simulink model "PMSM_Demo"  (R2019b)
settings: Solver=FixedStepDiscrete  StartTime=0.0  StopTime=Inf  FixedStep=1000e-6  RelTol=1e-3  EnableMultiTasking=on
PreLoadFcn:
  | run('PMSM_Demo_ini.m');
PostLoadFcn:
  | , if any(exist('dsrtsu_mdlpostloadfcn', 'file') ~= 0), dsrtsu_mdlpostloadfcn('Execute', bdroot); end,
InitFcn:
  | , if any(exist('rtifpga_mdlclblib', 'file') ~= 0), rtifpga_mdlclblib('Init', bdroot); end,
values from neighbouring files (symbols this model uses):
  Const_Id_Fieldweakening = 0    [PMSM_Demo_ini.m]
  Const_Ld_Stator = L    (= 0.0004)    [PMSM_Demo_ini.m]
  Const_Lq_Stator = L    (= 0.0004)    [PMSM_Demo_ini.m]
  Const_PolePairs = PolePairs    (= 4)    [PMSM_Demo_ini.m]
  Const_Psi = Psi    (= 0.017)    [PMSM_Demo_ini.m]
  PMSM_Ctrl_Ctrl_mode_SW = 3    [PMSM_Demo_ini.m]
  PMSM_Ctrl_fRS_Set = 0    [PMSM_Demo_ini.m]
  PMSM_Ctrl_i_d_Set = 0    [PMSM_Demo_ini.m]
  PMSM_Ctrl_i_d_Stroke = 0    [PMSM_Demo_ini.m]
  PMSM_Ctrl_i_q_Set = 0    [PMSM_Demo_ini.m]
  PMSM_Ctrl_i_q_Stroke = 0    [PMSM_Demo_ini.m]
  PMSM_Ctrl_Ki_id = KI_i    (= 3595.02029348)    [PMSM_Demo_ini.m]
  PMSM_Ctrl_Ki_iq = KI_i    (= 3595.02029348)    [PMSM_Demo_ini.m]
  PMSM_Ctrl_Ki_n = KI_n    (= 50.0861118327)    [PMSM_Demo_ini.m]
  PMSM_Ctrl_Kp_id = KP_i    (= 1.54995705396)    [PMSM_Demo_ini.m]
  PMSM_Ctrl_Kp_iq = KP_i    (= 1.54995705396)    [PMSM_Demo_ini.m]
  PMSM_Ctrl_Kp_n = KP_n    (= 0.0775235575931)    [PMSM_Demo_ini.m]
  PMSM_Ctrl_Limit_iq = IQ_MAX    (= 10.6)    [PMSM_Demo_ini.m]
  PMSM_Ctrl_load_torque = 0    [PMSM_Demo_ini.m]
  PMSM_Ctrl_n_Limit = N_MAX    (= 3000)    [PMSM_Demo_ini.m]
  PMSM_Ctrl_n_Set = 0    [PMSM_Demo_ini.m]
  PMSM_Ctrl_n_Stroke = 0    [PMSM_Demo_ini.m]
  PMSM_Ctrl_Pos_Src = 1    [PMSM_Demo_ini.m]
  PMSM_Ctrl_TF_Id = TF_i    (= 7.95774715459e-05)    [PMSM_Demo_ini.m]
  PMSM_Ctrl_TF_Iq = TF_i    (= 7.95774715459e-05)    [PMSM_Demo_ini.m]
  PMSM_Ctrl_TF_n = TF_n    (= 0.00106103295395)    [PMSM_Demo_ini.m]
  PMSM_Ctrl_theta_offset = 0.5    [PMSM_Demo_ini.m]
  PMSM_Ctrl_v_d_Set = 0    [PMSM_Demo_ini.m]
  PMSM_Ctrl_V_DCLink_Limit = UD    (= 15)    [PMSM_Demo_ini.m]
  PMSM_Ctrl_v_q_Set = 0    [PMSM_Demo_ini.m]
  PMSM_Ctrl_Vel_Src = 4    [PMSM_Demo_ini.m]
  SW_Fieldweakening = 2    [PMSM_Demo_ini.m]
  T_PWM = 50e-6    (= 5e-05)    [PMSM_Demo_ini.m]
undefined symbols (not defined in the file or in its folder): clock, Newton, Raphson, rpm_to_rad, s
libraries: simulink x37, rti1202lib_adc_class1 x8, dsextras x4, rtiemclib x4, rti1202lib_dio_class1 x3, ASM_ElectricComponents_lib x2, ASM_Utils_lib x1, rti1202lib_base x1
(part 4 of 4)

== system PMSM_Demo/Control/Controller/PMSM_CONTROLLER/current_controller/current_transformation_disp ==
  in1 : Inport
  demux : Demux  Outputs=2
  transf : Subsystem
      settings: AttributesFormatString=clarke
  out1 : Outport  VectorParamsAs1DForOutWhenUnconnected=off
  out2 : Outport  Port=2  VectorParamsAs1DForOutWhenUnconnected=off
  wires:
  in1/1 -> transf/1(in)
  transf/1(out) -> demux/1
  demux/1 -> out1/1
  demux/2 -> out2/1

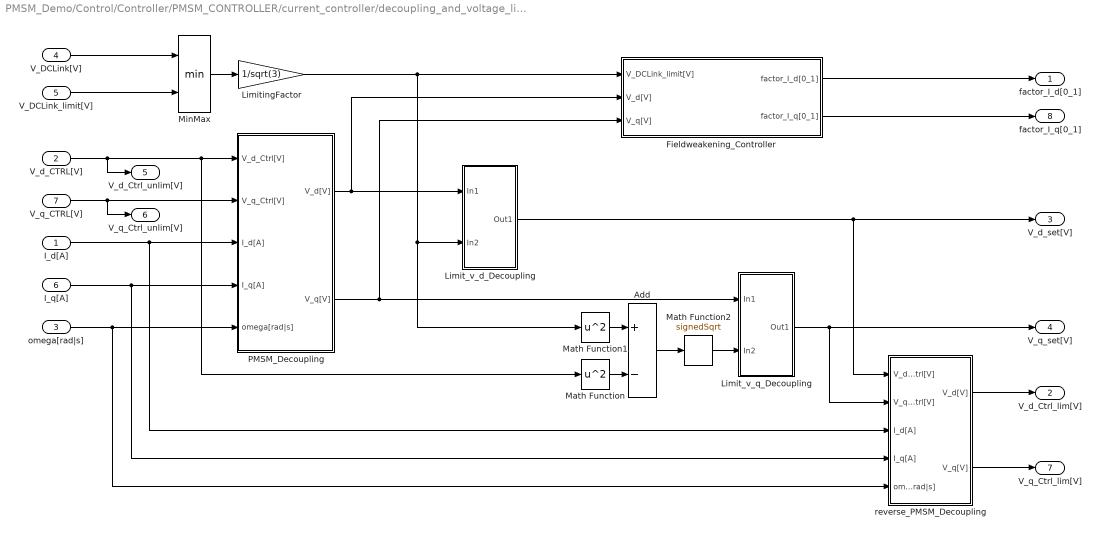
== system PMSM_Demo/Control/Controller/PMSM_CONTROLLER/current_controller/decoupling_and_voltage_limitation ==
  I_d[A] : Inport
  V_d_CTRL[V] : Inport  Port=2
  omega[rad|s] : Inport  Port=3
  V_DCLink[V] : Inport  Port=4
  V_DCLink_limit[V] : Inport  Port=5
  I_q[A] : Inport  Port=6
  V_q_CTRL[V] : Inport  Port=7
  Add : Sum  Inputs=+-
  Fieldweakening_Controller : Subsystem
  Limit_v_d_Decoupling : Subsystem
      mask Display: plot([0.15 0.85],[.5 .5],[.5 .5],[0.05 0.95],0.15+0.7*[0 .25 .75 1],0.05+0.9*[.25 .25 .75 .75]);
  Limit_v_q_Decoupling : Subsystem
      mask Display: plot([0.15 0.85],[.5 .5],[.5 .5],[0.05 0.95],0.15+0.7*[0 .25 .75 1],0.05+0.9*[.25 .25 .75 .75]);
  LimitingFactor : Gain  Gain=1/sqrt(3)
  Math Function : Math  Operator=square  SaturateOnIntegerOverflow=on
  Math Function1 : Math  Operator=square  SaturateOnIntegerOverflow=on
  Math Function2 : Sqrt  Operator=signedSqrt  AlgorithmType=Newton-Raphson  SaturateOnIntegerOverflow=on
  MinMax : MinMax  Inputs=2
  PMSM_Decoupling : Subsystem
  reverse_PMSM_Decoupling : Subsystem
  factor_I_d[0_1] : Outport  VectorParamsAs1DForOutWhenUnconnected=off
  V_d_Ctrl_lim[V] : Outport  Port=2  VectorParamsAs1DForOutWhenUnconnected=off
  V_d_set[V] : Outport  Port=3  VectorParamsAs1DForOutWhenUnconnected=off
  V_q_set[V] : Outport  Port=4  VectorParamsAs1DForOutWhenUnconnected=off
  V_d_Ctrl_unlim[V] : Outport  Port=5  VectorParamsAs1DForOutWhenUnconnected=off
  V_q_Ctrl_unlim[V] : Outport  Port=6  VectorParamsAs1DForOutWhenUnconnected=off
  V_q_Ctrl_lim[V] : Outport  Port=7  VectorParamsAs1DForOutWhenUnconnected=off
  factor_I_q[0_1] : Outport  Port=8  VectorParamsAs1DForOutWhenUnconnected=off
  wires:
  Fieldweakening_Controller/2(factor_I_q[0_1]) -> factor_I_q[0_1]/1
  Fieldweakening_Controller/1(factor_I_d[0_1]) -> factor_I_d[0_1]/1
  Math Function2/1 -> Limit_v_q_Decoupling/2(In2)
  V_DCLink_limit[V]/1 -> MinMax/2
  Limit_v_q_Decoupling/1(Out1) -> reverse_PMSM_Decoupling/2(V_q_Ctrl[V]), V_q_set[V]/1
  Limit_v_d_Decoupling/1(Out1) -> reverse_PMSM_Decoupling/1(V_d_Ctrl[V]), V_d_set[V]/1
  reverse_PMSM_Decoupling/2(V_q[V]) -> V_q_Ctrl_lim[V]/1
  reverse_PMSM_Decoupling/1(V_d[V]) -> V_d_Ctrl_lim[V]/1
  PMSM_Decoupling/2(V_q[V]) -> Limit_v_q_Decoupling/1(In1), Fieldweakening_Controller/3(V_q[V])
  Add/1 -> Math Function2/1
  Math Function/1 -> Add/2
  Math Function1/1 -> Add/1
  LimitingFactor/1 -> Math Function1/1, Limit_v_d_Decoupling/2(In2), Fieldweakening_Controller/1(V_DCLink_limit[V])
  omega[rad|s]/1 -> reverse_PMSM_Decoupling/5(omega[rad|s]), PMSM_Decoupling/5(omega[rad|s])
  PMSM_Decoupling/1(V_d[V]) -> Limit_v_d_Decoupling/1(In1), Fieldweakening_Controller/2(V_d[V])
  I_d[A]/1 -> reverse_PMSM_Decoupling/3(I_d[A]), PMSM_Decoupling/3(I_d[A])
  I_q[A]/1 -> reverse_PMSM_Decoupling/4(I_q[A]), PMSM_Decoupling/4(I_q[A])
  V_d_CTRL[V]/1 -> Math Function/1, PMSM_Decoupling/1(V_d_Ctrl[V]), V_d_Ctrl_unlim[V]/1
  V_q_CTRL[V]/1 -> PMSM_Decoupling/2(V_q_Ctrl[V]), V_q_Ctrl_unlim[V]/1
  V_DCLink[V]/1 -> MinMax/1
  MinMax/1 -> LimitingFactor/1

== system PMSM_Demo/Control/Controller/PMSM_CONTROLLER/current_controller/manip_i_d ==
  Factor_i_d[0_1] : Inport
  I_d_Set[A] : Inport  Port=2
  SW : Inport  Port=3
  Multiport Switch : MultiPortSwitch
  factor_id : Product  RndMeth=Zero
  Out1 : Outport  VectorParamsAs1DForOutWhenUnconnected=off
  wires:
  factor_id/1 -> Multiport Switch/2
  Factor_i_d[0_1]/1 -> factor_id/1
  Multiport Switch/1 -> Out1/1
  SW/1 -> Multiport Switch/1
  I_d_Set[A]/1 -> Multiport Switch/4, Multiport Switch/3, factor_id/2

== system PMSM_Demo/Control/Controller/PMSM_CONTROLLER/current_controller/manip_i_q ==
  SW : Inport
  I_q_Set[A] : Inport  Port=2
  Factor_i_q[0_1] : Inport  Port=3
  Multiport Switch : MultiPortSwitch
  factor_id : Product  RndMeth=Zero
  Out1 : Outport  VectorParamsAs1DForOutWhenUnconnected=off
  wires:
  factor_id/1 -> Multiport Switch/2
  Factor_i_q[0_1]/1 -> factor_id/1
  I_q_Set[A]/1 -> Multiport Switch/4, Multiport Switch/3, factor_id/2
  SW/1 -> Multiport Switch/1
  Multiport Switch/1 -> Out1/1

== system PMSM_Demo/Control/Controller/PMSM_CONTROLLER/i_set_source_SW/Limit_id_Set ==
  In1 : Inport
  In2 : Inport  Port=2
  Saturation Dynamic : simulink/Discontinuities/Saturation Dynamic  OutMin=[]  OutMax=[]  OutDataTypeStr=Inherit: Same as second input  OutDataType=sfix(16)  OutScaling=2^-10  DoSatur=off
  inv : Gain  Gain=-1
  Out1 : Outport  VectorParamsAs1DForOutWhenUnconnected=off
  wires:
  inv/1 -> Saturation Dynamic/3
  In2/1 -> Saturation Dynamic/1, inv/1
  In1/1 -> Saturation Dynamic/2
  Saturation Dynamic/1 -> Out1/1

== system PMSM_Demo/Control/Controller/PMSM_CONTROLLER/i_set_source_SW/Limit_iq_Set ==
  In1 : Inport
  In2 : Inport  Port=2
  Saturation Dynamic : simulink/Discontinuities/Saturation Dynamic  OutMin=[]  OutMax=[]  OutDataTypeStr=Inherit: Same as second input  OutDataType=sfix(16)  OutScaling=2^-10  DoSatur=off
  inv : Gain  Gain=-1
  Out1 : Outport  VectorParamsAs1DForOutWhenUnconnected=off
  wires:
  Saturation Dynamic/1 -> Out1/1
  In1/1 -> Saturation Dynamic/2
  In2/1 -> inv/1, Saturation Dynamic/1
  inv/1 -> Saturation Dynamic/3

== system PMSM_Demo/Control/Controller/PMSM_CONTROLLER/speed_controller/DISCRETE_PT1 ==
  Reset[0|1] : Inport
  In : Inport  Port=2
  K : Inport  Port=3
  T[s] : Inport  Port=4
  T_Sample[s] : Inport  Port=5
  1|FilterTime : Product  Inputs=*/  SaturateOnIntegerOverflow=on  InputSameDT=on  OutDataTypeStr=Inherit: Same as first input
  Proportional : Product  Inputs=**  SaturateOnIntegerOverflow=on  InputSameDT=on  OutDataTypeStr=Inherit: Same as first input
  Sum : Sum  Inputs=-+|  SaturateOnIntegerOverflow=on  InputSameDT=on  OutDataTypeStr=Inherit: Same as first input
  Unit Delay : UnitDelay  SampleTime=-1  HasFrameUpgradeWarning=on
  discrete_Integrator_Init : Subsystem  mask(DISCRETE_INTEGRATOR){upper_limit=upper_limit_int, lower_limit=lower_limit_int, ASMProperties=struct('Name','discrete_integrator','Version','1.0','Library','ASM_ElectricComponents_lib')}
      mask prompts: upper_limit "upper limit"; lower_limit "lower limit"
      mask help: (c) Copyright 2007, dSPACE GmbH. All rights reserved.
      mask Help: eval(['asm_modelhelp(gcbh)'])
  zero : Constant  Value=0  SampleTime=-1
  Out : Outport  VectorParamsAs1DForOutWhenUnconnected=off
  wires:
  In/1 -> Proportional/1
  Sum/1 -> discrete_Integrator_Init/2(In)
  K/1 -> Proportional/2
  Proportional/1 -> Sum/2
  discrete_Integrator_Init/1(Out) -> 1|FilterTime/1
  1|FilterTime/1 -> Out/1, Unit Delay/1
  Unit Delay/1 -> Sum/1
  T[s]/1 -> 1|FilterTime/2
  Reset[0|1]/1 -> discrete_Integrator_Init/1(Reset[0|1])
  T_Sample[s]/1 -> discrete_Integrator_Init/4(T_Sample[s])
  zero/1 -> discrete_Integrator_Init/3(Initial)

== system PMSM_Demo/Control/Controller/PMSM_CONTROLLER/speed_controller/DISCRETE_PT1_SET ==
  Reset[0|1] : Inport
  In : Inport  Port=2
  K : Inport  Port=3
  T[s] : Inport  Port=4
  T_Sample[s] : Inport  Port=5
  1|FilterTime : Product  Inputs=*/  SaturateOnIntegerOverflow=on  InputSameDT=on  OutDataTypeStr=Inherit: Same as first input
  Proportional : Product  Inputs=**  SaturateOnIntegerOverflow=on  InputSameDT=on  OutDataTypeStr=Inherit: Same as first input
  Sum : Sum  Inputs=-+|  SaturateOnIntegerOverflow=on  InputSameDT=on  OutDataTypeStr=Inherit: Same as first input
  Unit Delay : UnitDelay  SampleTime=-1  HasFrameUpgradeWarning=on
  discrete_Integrator_Init : Subsystem  mask(DISCRETE_INTEGRATOR){upper_limit=upper_limit_int, lower_limit=lower_limit_int, ASMProperties=struct('Name','discrete_integrator','Version','1.0','Library','ASM_ElectricComponents_lib')}
      mask prompts: upper_limit "upper limit"; lower_limit "lower limit"
      mask help: (c) Copyright 2007, dSPACE GmbH. All rights reserved.
      mask Help: eval(['asm_modelhelp(gcbh)'])
  zero : Constant  Value=0  SampleTime=-1
  Out : Outport  VectorParamsAs1DForOutWhenUnconnected=off
  wires:
  zero/1 -> discrete_Integrator_Init/3(Initial)
  T_Sample[s]/1 -> discrete_Integrator_Init/4(T_Sample[s])
  Reset[0|1]/1 -> discrete_Integrator_Init/1(Reset[0|1])
  T[s]/1 -> 1|FilterTime/2
  Unit Delay/1 -> Sum/1
  1|FilterTime/1 -> Unit Delay/1, Out/1
  discrete_Integrator_Init/1(Out) -> 1|FilterTime/1
  Proportional/1 -> Sum/2
  K/1 -> Proportional/2
  Sum/1 -> discrete_Integrator_Init/2(In)
  In/1 -> Proportional/1

== system PMSM_Demo/Control/Controller/PMSM_CONTROLLER/speed_controller/Limit_n_Set ==
  In1 : Inport
  In2 : Inport  Port=2
  Saturation Dynamic : simulink/Discontinuities/Saturation Dynamic  OutMin=[]  OutMax=[]  OutDataTypeStr=Inherit: Same as second input  OutDataType=sfix(16)  OutScaling=2^-10  DoSatur=off
  inv : Gain  Gain=-1
  Out1 : Outport  VectorParamsAs1DForOutWhenUnconnected=off
  wires:
  inv/1 -> Saturation Dynamic/3
  In2/1 -> Saturation Dynamic/1, inv/1
  In1/1 -> Saturation Dynamic/2
  Saturation Dynamic/1 -> Out1/1

== system PMSM_Demo/Control/Controller/PMSM_CONTROLLER/speed_controller/PI_CONTROLLER ==
  ActualValue : Inport
  RefValue : Inport  Port=2
  Kp : Inport  Port=3
  Ki : Inport  Port=4
  Limit_up : Inport  Port=5
  Limit_lo : Inport  Port=6
  T_Sample[s] : Inport  Port=7
  Product : Product  RndMeth=Zero
  Product1 : Product  RndMeth=Zero
  Product2 : Product  RndMeth=Zero
  Saturation Dynamic : simulink/Discontinuities/Saturation Dynamic  OutMin=[]  OutMax=[]  OutDataTypeStr=Inherit: Same as second input  OutDataType=sfix(16)  OutScaling=2^-10  DoSatur=off
  Sum : Sum  Inputs=+++  SaturateOnIntegerOverflow=on
  Sum1 : Sum  Inputs=+-  SaturateOnIntegerOverflow=on
  Sum2 : Sum  Inputs=-+|  SaturateOnIntegerOverflow=on
  Unit Delay : UnitDelay  SampleTime=-1  HasFrameUpgradeWarning=on
  y : Outport  VectorParamsAs1DForOutWhenUnconnected=off
  wires:
  Limit_lo/1 -> Saturation Dynamic/3
  Limit_up/1 -> Saturation Dynamic/1
  Sum/1 -> Saturation Dynamic/2
  Sum1/1 -> Product1/2, Product2/1  "error"
  RefValue/1 -> Sum1/1
  ActualValue/1 -> Sum1/2
  Product1/1 -> Sum/1, Sum2/1
  Product/1 -> Sum/2  "integral"
  Saturation Dynamic/1 -> Sum2/2, y/1
  Product2/1 -> Product/1
  Unit Delay/1 -> Sum/3
  Sum2/1 -> Unit Delay/1
  T_Sample[s]/1 -> Product/2
  Kp/1 -> Product1/1
  Ki/1 -> Product2/2

== system PMSM_Demo/Control/Controller/PMSM_CONTROLLER/speed_controller/SignalCollector ==
  n_Limit[rpm] : Inport
  n[rpm] : Inport  Port=2
  n_Set[rpm] : Inport  Port=3
  Bus Creator : BusCreator  Inputs=3
  SignalBus : Outport  VectorParamsAs1DForOutWhenUnconnected=off
  wires:
  n_Limit[rpm]/1 -> Bus Creator/3  "n_Limit[rpm]"
  Bus Creator/1 -> SignalBus/1  "SPEED_CONTROLLER"
  n_Set[rpm]/1 -> Bus Creator/2  "n_Set[rpm]"
  n[rpm]/1 -> Bus Creator/1  "n[rpm]"

== system PMSM_Demo/Control/Controller/PMSM_CONTROLLER/v_set_source_SW/Calc_Angle ==
  f_set[Hz] : Inport
  T_Sample[s] : Inport  Port=2
  DISCRETE_INTEGRATOR : Subsystem  mask(DISCRETE_INTEGRATOR){upper_limit=struct('v', 1e300), lower_limit=struct('v', -1e300), ASMProperties=struct('Name','DISCRETE_INTEGRATOR','Version','1.0','Library','ASM_ElectricComponents_lib')}
      mask prompts: upper_limit "upper limit"; lower_limit "lower limit"
      mask help: (c) Copyright 2007, dSPACE GmbH. All rights reserved.
      mask Help: eval(['asm_modelhelp(gcbh)'])
  Lim[0...2*pi] : Subsystem
  Reset[0|1] : Constant  Value=0
  "[rpm]2[rad|s]" : ASM_Utils_lib/UnitConversion/UnitConversion  Selection=rpm_to_rad/s
  torpm : Gain  Gain=60  SaturateOnIntegerOverflow=on  OutDataTypeStr=Inherit: Same as input  ParamDataTypeStr=Inherit: Same as input
  zero : Constant  Value=0
  theta[rad] : Outport  VectorParamsAs1DForOutWhenUnconnected=off
  wires:
  Lim[0...2*pi]/1(theta_lim) -> theta[rad]/1
  T_Sample[s]/1 -> DISCRETE_INTEGRATOR/4(T_Sample[s])
  torpm/1 -> "[rpm]2[rad|s]"/1
  Reset[0|1]/1 -> DISCRETE_INTEGRATOR/1(Reset[0|1])
  zero/1 -> DISCRETE_INTEGRATOR/3(Initial)
  DISCRETE_INTEGRATOR/1(Out) -> Lim[0...2*pi]/1(theta_unlim)
  f_set[Hz]/1 -> torpm/1
  "[rpm]2[rad|s]"/1 -> DISCRETE_INTEGRATOR/2(In)

== system PMSM_Demo/Control/Controller/PMSM_CONTROLLER/v_set_source_SW/Label_v_Stator[a;b;c][V] ==
  In : Inport
  Bus Creator : BusCreator  Inputs=3
  Demux : Demux  Outputs=3
  Out : Outport  VectorParamsAs1DForOutWhenUnconnected=off
  wires:
  In/1 -> Demux/1
  Bus Creator/1 -> Out/1
  Demux/1 -> Bus Creator/1  "V_a_Stator[V]"
  Demux/2 -> Bus Creator/2  "V_b_Stator[V]"
  Demux/3 -> Bus Creator/3  "V_c_Stator[V]"

== system PMSM_Demo/Control/Input/DISCRETE_PT1/discrete_Integrator_Init/only_rising_edge  ==
  In1 : Inport
  Compare To Constant1 : simulink/Logic and Bit Operations/Compare To Constant  relop===  const=0  OutDataTypeStr=uint8  ZeroCross=off
  Compare To Constant2 : simulink/Logic and Bit Operations/Compare To Constant  relop===  const=1  OutDataTypeStr=uint8  ZeroCross=off
  Logical Operator1 : Logic  AllPortsSameDT=off  OutDataTypeStr=boolean
  Unit Delay2 : UnitDelay  SampleTime=-1  HasFrameUpgradeWarning=on
  Out1 : Outport  VectorParamsAs1DForOutWhenUnconnected=off
  wires:
  Logical Operator1/1 -> Out1/1
  Compare To Constant2/1 -> Logical Operator1/2
  Compare To Constant1/1 -> Logical Operator1/1
  In1/1 -> Compare To Constant2/1, Unit Delay2/1
  Unit Delay2/1 -> Compare To Constant1/1

== system PMSM_Demo/RTI Data/RTI Data Store/RTI Data Store/RTI Data Store/RTI Data Store ==

== system PMSM_Demo/Control/Controller/PMSM_CONTROLLER/current_controller/DISCRETE_PT1/discrete_Integrator_Init ==
  Reset[0|1] : Inport
  In : Inport  Port=2
  Initial : Inport  Port=3
  T_Sample[s] : Inport  Port=4
  Add : Sum  Inputs=+++
  Compare To Constant : simulink/Logic and Bit Operations/Compare To Constant  relop===  const=0  OutDataTypeStr=uint8  ZeroCross=off
  Constant1 : Constant  Value=0
  Constant2 : Constant  Value=0
  Logical Operator : Logic  Operator=OR  AllPortsSameDT=off  OutDataTypeStr=boolean
  Product : Product  RndMeth=Zero
  Saturation : simulink/Discontinuities/Saturation Dynamic  OutMin=[]  OutMax=[]  OutDataTypeStr=Inherit: Same as second input  OutDataType=sfix(16)  OutScaling=2^-10  DoSatur=off
  Switch1 : Switch  Threshold=0.5
  Switch2 : Switch  Threshold=0.5
  Unit Delay : UnitDelay  SampleTime=-1  HasFrameUpgradeWarning=on
  Unit Delay1 : UnitDelay  SampleTime=-1  HasFrameUpgradeWarning=on
  lower_limit : Constant  Value=lower_limit.v
  "only_rising_edge " : Subsystem
  upper_limit : Constant  Value=upper_limit.v
  Out : Outport  VectorParamsAs1DForOutWhenUnconnected=off
  wires:
  Compare To Constant/1 -> Logical Operator/1
  Logical Operator/1 -> Switch1/2
  Unit Delay1/1 -> Compare To Constant/1
  "only_rising_edge "/1(Out1) -> Switch2/2, Logical Operator/2
  Constant1/1 -> Switch1/3
  Initial/1 -> Switch1/1
  Switch1/1 -> Add/1
  Unit Delay/1 -> Switch2/3
  Switch2/1 -> Add/3
  Constant2/1 -> Switch2/1
  In/1 -> Product/2
  Reset[0|1]/1 -> "only_rising_edge "/1(In1)
  Product/1 -> Add/2
  T_Sample[s]/1 -> Unit Delay1/1, Product/1
  Add/1 -> Saturation/2
  Saturation/1 -> Out/1, Unit Delay/1
  upper_limit/1 -> Saturation/1
  lower_limit/1 -> Saturation/3

== system PMSM_Demo/Control/Controller/PMSM_CONTROLLER/current_controller/DISCRETE_PT2/discrete_Integrator_Init ==
  Reset[0|1] : Inport
  In : Inport  Port=2
  Initial : Inport  Port=3
  T_Sample[s] : Inport  Port=4
  Add : Sum  Inputs=+++
  Compare To Constant : simulink/Logic and Bit Operations/Compare To Constant  relop===  const=0  OutDataTypeStr=uint8  ZeroCross=off
  Constant1 : Constant  Value=0
  Constant2 : Constant  Value=0
  Logical Operator : Logic  Operator=OR  AllPortsSameDT=off  OutDataTypeStr=boolean
  Product : Product  RndMeth=Zero
  Saturation : simulink/Discontinuities/Saturation Dynamic  OutMin=[]  OutMax=[]  OutDataTypeStr=Inherit: Same as second input  OutDataType=sfix(16)  OutScaling=2^-10  DoSatur=off
  Switch1 : Switch  Threshold=0.5
  Switch2 : Switch  Threshold=0.5
  Unit Delay : UnitDelay  SampleTime=-1  HasFrameUpgradeWarning=on
  Unit Delay1 : UnitDelay  SampleTime=-1  HasFrameUpgradeWarning=on
  lower_limit : Constant  Value=lower_limit.v
  "only_rising_edge " : Subsystem
  upper_limit : Constant  Value=upper_limit.v
  Out : Outport  VectorParamsAs1DForOutWhenUnconnected=off
  wires:
  lower_limit/1 -> Saturation/3
  upper_limit/1 -> Saturation/1
  Saturation/1 -> Unit Delay/1, Out/1
  Add/1 -> Saturation/2
  T_Sample[s]/1 -> Product/1, Unit Delay1/1
  Product/1 -> Add/2
  Reset[0|1]/1 -> "only_rising_edge "/1(In1)
  In/1 -> Product/2
  Constant2/1 -> Switch2/1
  Switch2/1 -> Add/3
  Unit Delay/1 -> Switch2/3
  Switch1/1 -> Add/1
  Initial/1 -> Switch1/1
  Constant1/1 -> Switch1/3
  "only_rising_edge "/1(Out1) -> Logical Operator/2, Switch2/2
  Unit Delay1/1 -> Compare To Constant/1
  Logical Operator/1 -> Switch1/2
  Compare To Constant/1 -> Logical Operator/1

== system PMSM_Demo/Control/Controller/PMSM_CONTROLLER/current_controller/current transformation/transf ==
  in : Inport
  Demux : Demux  Outputs=[3 1]
  Demux1 : Demux  Outputs=2
  Gain1 : Gain  Gain=[[2/3 -1/3 -1/3]*transffactor;[0 sqrt(3)/3 -sqrt(3)/3]*transffactor]  Multiplication=Matrix(K*u)  SaturateOnIntegerOverflow=on  OutDataTypeStr=Inherit: Same as input  ParamDataTypeStr=Inherit: Same as input
  Mux : Mux  Inputs=2
  Product{1..4} (4 alike) : Product  SaturateOnIntegerOverflow=on  OutDataTypeStr=Inherit: Same as first input
  Sum : Sum  SaturateOnIntegerOverflow=on
  Sum1 : Sum  SaturateOnIntegerOverflow=on
  cos : Fcn  Expr=cos(u)
  inv : Gain  Gain=-1  SaturateOnIntegerOverflow=on  OutDataTypeStr=Inherit: Same as input  ParamDataTypeStr=Inherit: Same as input
  sin : Fcn  Expr=sin(u)
  out : Outport  VectorParamsAs1DForOutWhenUnconnected=off
  wires:
  Mux/1 -> out/1
  in/1 -> Demux/1
  Demux/1 -> Gain1/1
  sin/1 -> inv/1, Product2/2
  Product3/1 -> Sum/1
  Product4/1 -> Sum/2
  Product2/1 -> Sum1/2
  Product1/1 -> Sum1/1
  Sum1/1 -> Mux/1
  Sum/1 -> Mux/2
  Demux/2 -> sin/1, cos/1
  cos/1 -> Product1/2, Product4/2
  inv/1 -> Product3/2
  Demux1/1 -> Product1/1, Product3/1
  Gain1/1 -> Demux1/1
  Demux1/2 -> Product2/1, Product4/1

== system PMSM_Demo/Control/Controller/PMSM_CONTROLLER/current_controller/current_transformation_disp/transf ==
  in : Inport
  Gain1 : Gain  Gain=[[2/3 -1/3 -1/3]*1;[0 sqrt(3)/3 -sqrt(3)/3]*1]  Multiplication=Matrix(K*u)  SaturateOnIntegerOverflow=on  OutDataTypeStr=Inherit: Same as input  ParamDataTypeStr=Inherit: Same as input
  out : Outport  VectorParamsAs1DForOutWhenUnconnected=off
  wires:
  in/1 -> Gain1/1
  Gain1/1 -> out/1

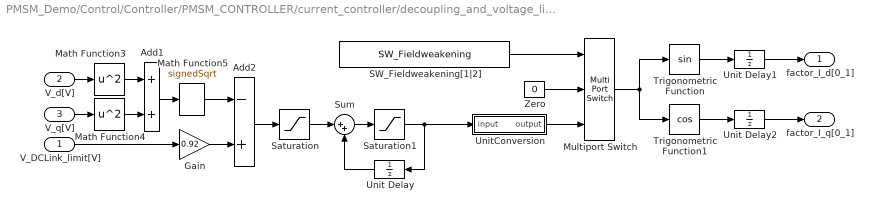
== system PMSM_Demo/Control/Controller/PMSM_CONTROLLER/current_controller/decoupling_and_voltage_limitation/Fieldweakening_Controller ==
  V_DCLink_limit[V] : Inport
  V_d[V] : Inport  Port=2
  V_q[V] : Inport  Port=3
  Add1 : Sum
  Add2 : Sum  Inputs=-+
  Gain : Gain  Gain=0.92
  Math Function3 : Math  Operator=square  SaturateOnIntegerOverflow=on
  Math Function4 : Math  Operator=square  SaturateOnIntegerOverflow=on
  Math Function5 : Sqrt  Operator=signedSqrt  AlgorithmType=Newton-Raphson  SaturateOnIntegerOverflow=on
  Multiport Switch : MultiPortSwitch  Inputs=2
  SW_Fieldweakening[1|2] : Constant  Value=SW_Fieldweakening
  Saturation : Saturate  UpperLimit=0.2  LowerLimit=-0.2
  Saturation1 : Saturate  UpperLimit=0  LowerLimit=-50
  Sum : Sum  Inputs=|++
  Trigonometric Function : Trigonometry
  Trigonometric Function1 : Trigonometry  Operator=cos
  Unit Delay : UnitDelay  SampleTime=-1  HasFrameUpgradeWarning=on
  Unit Delay1 : UnitDelay  SampleTime=-1  HasFrameUpgradeWarning=on
  Unit Delay2 : UnitDelay  SampleTime=-1  HasFrameUpgradeWarning=on
  UnitConversion : Subsystem  mask{Selection=deg_to_rad}
      mask prompts: Selection "Conversion:"
      mask init:
      | if(~exist('DS_CONTROLDESK_EVALUATION'))
      |     
      |   switch Selection
      |       
      |     case 'none'
      |       Offset = 0; Gain = 1; Unit1 = ''; Unit2 = '';      
      |     case 'bar_to_Pa'
      |       Offset = 0; Gain = 100000; Unit1 = 'bar'; Unit2 = 'Pa';
      |     case 'rad_to_deg'
      |       Offset = 0; Gain = 180/pi; Unit1 = 'rad'; Unit2 = 'deg';
      |     case 'deg_to_rad'
      |       Offset = 0; Gain = pi/180; Unit1 = 'deg'; Unit2 = 'rad';
      |     case 'degC_to_K'
      |       Offset = 273; Gain = 1; Unit1 = 'degC'; Unit2 = 'K';
      |     case 'K_to_degC'
      |       Offset = -273; Gain = 1; Unit1 = 'K'; Unit2 = 'degC';      
      |     case 'km/h_to_m/s'
      |       Offset = 0; Gain = 1/3.6; Unit1 = 'km|h'; Unit2 = 'm|s';
      |     case 'kg/h_to_kg/s'
      |       Offset = 0; Gain = 1/3600; Unit1 = 'kg|h'; Unit2 = 'kg|s';
      |     case 'kg/s_to_kg/h'
      |       Offset = 0; Gain = 3600; Unit1 = 'kg|s'; Unit2 = 'kg|h';
      |     case 'm/s_to_km/h'
      |       Offset = 0; Gain = 3.6; Unit1 = 'm|s'; Unit2 = 'km|h';
      |     case 'mm_to_m'
      |       Offset = 0; Gain = 1/1000; Unit1 = 'mm'; Unit2 = 'm';
      |     case 'mm_to_cm'
      |       Offset = 0; Gain = 1/10; Unit1 = 'mm'; Unit2 = 'cm';
      |     case 'm_to_mm'
      |       Offset = 0; Gain = 1000; Unit1 = 'm'; Unit2 = 'mm';
      |     case 'm_to_cm'
      |       Offset = 0; Gain = 100; Unit1 = 'm'; Unit2 = 'cm';
      |     case 'Pa_to_bar'
      |       Offset = 0; Gain = 1/100000; Unit1 = 'Pa'; Unit2 = 'bar';
      |     case 'rad/s_to_rpm'
      |       Offset = 0; Gain = 30/pi; Unit1 = 'rad|s'; Unit2 = 'rpm';
      |     case 'rpm_to_rad/s'
      |        Offset = 0; Gain = pi/30; Unit1 = 'rpm'; Unit2 = 'rad|s';
      |     case 'rpm_to_deg/s'
      |        Offset = 0; Gain = 6; Unit1 = 'rpm'; Unit2 = 'deg|s'; 
      |     case 'deg/s_to_rpm'
      |        Offset = 0; Gain = 1/6; Unit1 = 'deg|s'; Unit2 = 'rpm'; 
      |     case '%_to_[0_1]'
      |       Offset = 0; Gain = 0.01; Unit1 = '%'; Unit2 = '0_1';
      |     case '[0_1]_to_%'
      |       Offset = 0; Gain = 100; Unit1 = '0_1'; Unit2 = '%';
      |     otherwise
      |       Offset = 0; Gain = 1; Unit1 = 'Error'; Unit2 = 'Error';
      |       
      |  
      |   end     
      | end
      mask TypeOptions Selection: none | bar_to_Pa | rad_to_deg | deg_to_rad | degC_to_K | K_to_degC | km/h_to_m/s | kg/h_to_kg/s | kg/s_to_kg/h | m/s_to_km/h | mm_to_m | mm_to_cm | m_to_mm | m_to_cm | Pa_to_bar | rad/s_to_rpm | rpm_to_rad/s | rpm_to_deg/s | deg/s_to_rpm | %_to_[0_1] | [0_1]_to_%
      mask Display:
      | port_label('input',1,['[', Unit1, ']'])
      | port_label('output',1, ['[', Unit2, ']'])
  Zero : Constant  Value=0
  factor_I_d[0_1] : Outport  VectorParamsAs1DForOutWhenUnconnected=off
  factor_I_q[0_1] : Outport  Port=2  VectorParamsAs1DForOutWhenUnconnected=off
  wires:
  Zero/1 -> Multiport Switch/2
  SW_Fieldweakening[1|2]/1 -> Multiport Switch/1
  Multiport Switch/1 -> Trigonometric Function1/1, Trigonometric Function/1
  UnitConversion/1(output) -> Multiport Switch/3
  V_DCLink_limit[V]/1 -> Gain/1
  V_q[V]/1 -> Math Function4/1
  V_d[V]/1 -> Math Function3/1
  Math Function3/1 -> Add1/1
  Math Function4/1 -> Add1/2
  Add1/1 -> Math Function5/1
  Math Function5/1 -> Add2/1
  Add2/1 -> Saturation/1
  Saturation/1 -> Sum/1
  Unit Delay/1 -> Sum/2
  Sum/1 -> Saturation1/1
  Trigonometric Function1/1 -> Unit Delay2/1
  Trigonometric Function/1 -> Unit Delay1/1
  Saturation1/1 -> UnitConversion/1(input), Unit Delay/1
  Unit Delay1/1 -> factor_I_d[0_1]/1
  Unit Delay2/1 -> factor_I_q[0_1]/1
  Gain/1 -> Add2/2

== system PMSM_Demo/Control/Controller/PMSM_CONTROLLER/current_controller/decoupling_and_voltage_limitation/Limit_v_d_Decoupling ==
  In1 : Inport
  In2 : Inport  Port=2
  Saturation Dynamic : simulink/Discontinuities/Saturation Dynamic  OutMin=[]  OutMax=[]  OutDataTypeStr=Inherit: Same as second input  OutDataType=sfix(16)  OutScaling=2^-10  DoSatur=off
  inv : Gain  Gain=-1
  Out1 : Outport  VectorParamsAs1DForOutWhenUnconnected=off
  wires:
  inv/1 -> Saturation Dynamic/3
  In2/1 -> Saturation Dynamic/1, inv/1
  In1/1 -> Saturation Dynamic/2
  Saturation Dynamic/1 -> Out1/1

== system PMSM_Demo/Control/Controller/PMSM_CONTROLLER/current_controller/decoupling_and_voltage_limitation/Limit_v_q_Decoupling ==
  In1 : Inport
  In2 : Inport  Port=2
  Saturation Dynamic : simulink/Discontinuities/Saturation Dynamic  OutMin=[]  OutMax=[]  OutDataTypeStr=Inherit: Same as second input  OutDataType=sfix(16)  OutScaling=2^-10  DoSatur=off
  inv : Gain  Gain=-1
  Out1 : Outport  VectorParamsAs1DForOutWhenUnconnected=off
  wires:
  inv/1 -> Saturation Dynamic/3
  In2/1 -> Saturation Dynamic/1, inv/1
  In1/1 -> Saturation Dynamic/2
  Saturation Dynamic/1 -> Out1/1

== system PMSM_Demo/Control/Controller/PMSM_CONTROLLER/current_controller/decoupling_and_voltage_limitation/PMSM_Decoupling ==
  V_d_Ctrl[V] : Inport
  V_q_Ctrl[V] : Inport  Port=2
  I_d[A] : Inport  Port=3
  I_q[A] : Inport  Port=4
  omega[rad|s] : Inport  Port=5
  Const_Lsd[H] : Gain  Gain=Const_Ld  SaturateOnIntegerOverflow=on  OutDataTypeStr=Inherit: Same as input  ParamDataTypeStr=Inherit: Same as input
  Const_Lsq[H] : Gain  Gain=Const_Lq  SaturateOnIntegerOverflow=on  OutDataTypeStr=Inherit: Same as input  ParamDataTypeStr=Inherit: Same as input
  Const_Psi[Wb] : Gain  Gain=Const_Psi  SaturateOnIntegerOverflow=on  OutDataTypeStr=Inherit: Same as input  ParamDataTypeStr=Inherit: Same as input
  Product : Product  SaturateOnIntegerOverflow=on  OutDataTypeStr=Inherit: Same as first input
  Product1 : Product  SaturateOnIntegerOverflow=on  OutDataTypeStr=Inherit: Same as first input
  Sum1 : Sum  Inputs=|++  SaturateOnIntegerOverflow=on
  Sum3 : Sum  Inputs=|+-  SaturateOnIntegerOverflow=on
  Sum4 : Sum  Inputs=|++  SaturateOnIntegerOverflow=on
  V_d[V] : Outport  VectorParamsAs1DForOutWhenUnconnected=off
  V_q[V] : Outport  Port=2  VectorParamsAs1DForOutWhenUnconnected=off
  wires:
  I_q[A]/1 -> Product/1
  omega[rad|s]/1 -> Const_Psi[Wb]/1, Product1/1, Product/2
  Const_Lsd[H]/1 -> Sum3/2
  Sum3/1 -> V_d[V]/1
  Sum4/1 -> V_q[V]/1
  Product1/1 -> Const_Lsq[H]/1
  Const_Lsq[H]/1 -> Sum1/2
  I_d[A]/1 -> Product1/2
  V_q_Ctrl[V]/1 -> Sum1/1
  Product/1 -> Const_Lsd[H]/1
  V_d_Ctrl[V]/1 -> Sum3/1
  Const_Psi[Wb]/1 -> Sum4/2
  Sum1/1 -> Sum4/1

== system PMSM_Demo/Control/Controller/PMSM_CONTROLLER/current_controller/decoupling_and_voltage_limitation/reverse_PMSM_Decoupling ==
  V_d_Ctrl[V] : Inport
  V_q_Ctrl[V] : Inport  Port=2
  I_d[A] : Inport  Port=3
  I_q[A] : Inport  Port=4
  omega[rad|s] : Inport  Port=5
  Const_Lsd[H] : Gain  Gain=Const_Ld  SaturateOnIntegerOverflow=on  OutDataTypeStr=Inherit: Same as input  ParamDataTypeStr=Inherit: Same as input
  Const_Lsq[H] : Gain  Gain=Const_Lq  SaturateOnIntegerOverflow=on  OutDataTypeStr=Inherit: Same as input  ParamDataTypeStr=Inherit: Same as input
  Const_Psi[Wb] : Gain  Gain=Const_Psi  SaturateOnIntegerOverflow=on  OutDataTypeStr=Inherit: Same as input  ParamDataTypeStr=Inherit: Same as input
  Product : Product  SaturateOnIntegerOverflow=on  OutDataTypeStr=Inherit: Same as first input
  Product1 : Product  SaturateOnIntegerOverflow=on  OutDataTypeStr=Inherit: Same as first input
  Sum1 : Sum  Inputs=|+-  SaturateOnIntegerOverflow=on
  Sum3 : Sum  Inputs=|++  SaturateOnIntegerOverflow=on
  Sum4 : Sum  Inputs=|+-  SaturateOnIntegerOverflow=on
  V_d[V] : Outport  VectorParamsAs1DForOutWhenUnconnected=off
  V_q[V] : Outport  Port=2  VectorParamsAs1DForOutWhenUnconnected=off
  wires:
  I_q[A]/1 -> Product/1
  omega[rad|s]/1 -> Const_Psi[Wb]/1, Product1/1, Product/2
  Const_Lsd[H]/1 -> Sum3/2
  Sum3/1 -> V_d[V]/1
  Sum4/1 -> V_q[V]/1
  Product1/1 -> Const_Lsq[H]/1
  Const_Lsq[H]/1 -> Sum1/2
  I_d[A]/1 -> Product1/2
  V_q_Ctrl[V]/1 -> Sum1/1
  Product/1 -> Const_Lsd[H]/1
  V_d_Ctrl[V]/1 -> Sum3/1
  Const_Psi[Wb]/1 -> Sum4/2
  Sum1/1 -> Sum4/1

== system PMSM_Demo/Control/Controller/PMSM_CONTROLLER/speed_controller/DISCRETE_PT1/discrete_Integrator_Init ==
  Reset[0|1] : Inport
  In : Inport  Port=2
  Initial : Inport  Port=3
  T_Sample[s] : Inport  Port=4
  Add : Sum  Inputs=+++
  Compare To Constant : simulink/Logic and Bit Operations/Compare To Constant  relop===  const=0  OutDataTypeStr=uint8  ZeroCross=off
  Constant1 : Constant  Value=0
  Constant2 : Constant  Value=0
  Logical Operator : Logic  Operator=OR  AllPortsSameDT=off  OutDataTypeStr=boolean
  Product : Product  RndMeth=Zero
  Saturation : simulink/Discontinuities/Saturation Dynamic  OutMin=[]  OutMax=[]  OutDataTypeStr=Inherit: Same as second input  OutDataType=sfix(16)  OutScaling=2^-10  DoSatur=off
  Switch1 : Switch  Threshold=0.5
  Switch2 : Switch  Threshold=0.5
  Unit Delay : UnitDelay  SampleTime=-1  HasFrameUpgradeWarning=on
  Unit Delay1 : UnitDelay  SampleTime=-1  HasFrameUpgradeWarning=on
  lower_limit : Constant  Value=lower_limit.v
  "only_rising_edge " : Subsystem
  upper_limit : Constant  Value=upper_limit.v
  Out : Outport  VectorParamsAs1DForOutWhenUnconnected=off
  wires:
  Compare To Constant/1 -> Logical Operator/1
  Logical Operator/1 -> Switch1/2
  Unit Delay1/1 -> Compare To Constant/1
  "only_rising_edge "/1(Out1) -> Switch2/2, Logical Operator/2
  Constant1/1 -> Switch1/3
  Initial/1 -> Switch1/1
  Switch1/1 -> Add/1
  Unit Delay/1 -> Switch2/3
  Switch2/1 -> Add/3
  Constant2/1 -> Switch2/1
  In/1 -> Product/2
  Reset[0|1]/1 -> "only_rising_edge "/1(In1)
  Product/1 -> Add/2
  T_Sample[s]/1 -> Unit Delay1/1, Product/1
  Add/1 -> Saturation/2
  Saturation/1 -> Out/1, Unit Delay/1
  upper_limit/1 -> Saturation/1
  lower_limit/1 -> Saturation/3

== system PMSM_Demo/Control/Controller/PMSM_CONTROLLER/speed_controller/DISCRETE_PT1_SET/discrete_Integrator_Init ==
  Reset[0|1] : Inport
  In : Inport  Port=2
  Initial : Inport  Port=3
  T_Sample[s] : Inport  Port=4
  Add : Sum  Inputs=+++
  Compare To Constant : simulink/Logic and Bit Operations/Compare To Constant  relop===  const=0  OutDataTypeStr=uint8  ZeroCross=off
  Constant1 : Constant  Value=0
  Constant2 : Constant  Value=0
  Logical Operator : Logic  Operator=OR  AllPortsSameDT=off  OutDataTypeStr=boolean
  Product : Product  RndMeth=Zero
  Saturation : simulink/Discontinuities/Saturation Dynamic  OutMin=[]  OutMax=[]  OutDataTypeStr=Inherit: Same as second input  OutDataType=sfix(16)  OutScaling=2^-10  DoSatur=off
  Switch1 : Switch  Threshold=0.5
  Switch2 : Switch  Threshold=0.5
  Unit Delay : UnitDelay  SampleTime=-1  HasFrameUpgradeWarning=on
  Unit Delay1 : UnitDelay  SampleTime=-1  HasFrameUpgradeWarning=on
  lower_limit : Constant  Value=lower_limit.v
  "only_rising_edge " : Subsystem
  upper_limit : Constant  Value=upper_limit.v
  Out : Outport  VectorParamsAs1DForOutWhenUnconnected=off
  wires:
  lower_limit/1 -> Saturation/3
  upper_limit/1 -> Saturation/1
  Saturation/1 -> Unit Delay/1, Out/1
  Add/1 -> Saturation/2
  T_Sample[s]/1 -> Product/1, Unit Delay1/1
  Product/1 -> Add/2
  Reset[0|1]/1 -> "only_rising_edge "/1(In1)
  In/1 -> Product/2
  Constant2/1 -> Switch2/1
  Switch2/1 -> Add/3
  Unit Delay/1 -> Switch2/3
  Switch1/1 -> Add/1
  Initial/1 -> Switch1/1
  Constant1/1 -> Switch1/3
  "only_rising_edge "/1(Out1) -> Logical Operator/2, Switch2/2
  Unit Delay1/1 -> Compare To Constant/1
  Logical Operator/1 -> Switch1/2
  Compare To Constant/1 -> Logical Operator/1

== system PMSM_Demo/Control/Controller/PMSM_CONTROLLER/v_set_source_SW/Calc_Angle/DISCRETE_INTEGRATOR ==
  Reset[0|1] : Inport
  In : Inport  Port=2
  Initial : Inport  Port=3
  T_Sample[s] : Inport  Port=4
  Add : Sum  Inputs=+++
  Compare To Constant : simulink/Logic and Bit Operations/Compare To Constant  relop===  const=0  OutDataTypeStr=uint8  ZeroCross=off
  Constant1 : Constant  Value=0
  Constant2 : Constant  Value=0
  Logical Operator : Logic  Operator=OR  AllPortsSameDT=off  OutDataTypeStr=boolean
  Product : Product  RndMeth=Zero
  Saturation : simulink/Discontinuities/Saturation Dynamic  OutMin=[]  OutMax=[]  OutDataTypeStr=Inherit: Same as second input  OutDataType=sfix(16)  OutScaling=2^-10  DoSatur=off
  Switch1 : Switch  Threshold=0.5
  Switch2 : Switch  Threshold=0.5
  Unit Delay : UnitDelay  SampleTime=-1  HasFrameUpgradeWarning=on
  Unit Delay1 : UnitDelay  SampleTime=-1  HasFrameUpgradeWarning=on
  lower_limit : Constant  Value=lower_limit.v
  "only_rising_edge " : Subsystem
  upper_limit : Constant  Value=upper_limit.v
  Out : Outport  VectorParamsAs1DForOutWhenUnconnected=off
  wires:
  Compare To Constant/1 -> Logical Operator/1
  Logical Operator/1 -> Switch1/2
  Unit Delay1/1 -> Compare To Constant/1
  "only_rising_edge "/1(Out1) -> Switch2/2, Logical Operator/2
  Constant1/1 -> Switch1/3
  Initial/1 -> Switch1/1
  Switch1/1 -> Add/1
  Unit Delay/1 -> Switch2/3
  Switch2/1 -> Add/3
  Constant2/1 -> Switch2/1
  In/1 -> Product/2
  Reset[0|1]/1 -> "only_rising_edge "/1(In1)
  Product/1 -> Add/2
  T_Sample[s]/1 -> Unit Delay1/1, Product/1
  Add/1 -> Saturation/2
  Saturation/1 -> Out/1, Unit Delay/1
  upper_limit/1 -> Saturation/1
  lower_limit/1 -> Saturation/3

== system PMSM_Demo/Control/Controller/PMSM_CONTROLLER/v_set_source_SW/Calc_Angle/Lim[0...2*pi] ==
  theta_unlim : Inport
  Constant2 : Constant  Value=2*pi
  Math Function1 : Math  Operator=mod  SaturateOnIntegerOverflow=on
  theta_lim : Outport  VectorParamsAs1DForOutWhenUnconnected=off
  wires:
  Constant2/1 -> Math Function1/2
  Math Function1/1 -> theta_lim/1
  theta_unlim/1 -> Math Function1/1

== system PMSM_Demo/Control/Controller/PMSM_CONTROLLER/current_controller/DISCRETE_PT1/discrete_Integrator_Init/only_rising_edge  ==
  In1 : Inport
  Compare To Constant1 : simulink/Logic and Bit Operations/Compare To Constant  relop===  const=0  OutDataTypeStr=uint8  ZeroCross=off
  Compare To Constant2 : simulink/Logic and Bit Operations/Compare To Constant  relop===  const=1  OutDataTypeStr=uint8  ZeroCross=off
  Logical Operator1 : Logic  AllPortsSameDT=off  OutDataTypeStr=boolean
  Unit Delay2 : UnitDelay  SampleTime=-1  HasFrameUpgradeWarning=on
  Out1 : Outport  VectorParamsAs1DForOutWhenUnconnected=off
  wires:
  Logical Operator1/1 -> Out1/1
  Compare To Constant2/1 -> Logical Operator1/2
  Compare To Constant1/1 -> Logical Operator1/1
  In1/1 -> Compare To Constant2/1, Unit Delay2/1
  Unit Delay2/1 -> Compare To Constant1/1

== system PMSM_Demo/Control/Controller/PMSM_CONTROLLER/current_controller/DISCRETE_PT2/discrete_Integrator_Init/only_rising_edge  ==
  In1 : Inport
  Compare To Constant1 : simulink/Logic and Bit Operations/Compare To Constant  relop===  const=0  OutDataTypeStr=uint8  ZeroCross=off
  Compare To Constant2 : simulink/Logic and Bit Operations/Compare To Constant  relop===  const=1  OutDataTypeStr=uint8  ZeroCross=off
  Logical Operator1 : Logic  AllPortsSameDT=off  OutDataTypeStr=boolean
  Unit Delay2 : UnitDelay  SampleTime=-1  HasFrameUpgradeWarning=on
  Out1 : Outport  VectorParamsAs1DForOutWhenUnconnected=off
  wires:
  Unit Delay2/1 -> Compare To Constant1/1
  In1/1 -> Unit Delay2/1, Compare To Constant2/1
  Compare To Constant1/1 -> Logical Operator1/1
  Compare To Constant2/1 -> Logical Operator1/2
  Logical Operator1/1 -> Out1/1

== system PMSM_Demo/Control/Controller/PMSM_CONTROLLER/current_controller/decoupling_and_voltage_limitation/Fieldweakening_Controller/UnitConversion ==
  input : Inport
  Gain : Gain  Gain=Gain  SaturateOnIntegerOverflow=on  OutDataTypeStr=Inherit: Same as input  ParamDataTypeStr=Inherit: Same as input
  Offset : Constant  Value=Offset
  Sum : Sum  Inputs=|++  SaturateOnIntegerOverflow=on
  output : Outport  VectorParamsAs1DForOutWhenUnconnected=off
  wires:
  Sum/1 -> output/1
  Offset/1 -> Sum/2
  Gain/1 -> Sum/1
  input/1 -> Gain/1

== system PMSM_Demo/Control/Controller/PMSM_CONTROLLER/speed_controller/DISCRETE_PT1/discrete_Integrator_Init/only_rising_edge  ==
  In1 : Inport
  Compare To Constant1 : simulink/Logic and Bit Operations/Compare To Constant  relop===  const=0  OutDataTypeStr=uint8  ZeroCross=off
  Compare To Constant2 : simulink/Logic and Bit Operations/Compare To Constant  relop===  const=1  OutDataTypeStr=uint8  ZeroCross=off
  Logical Operator1 : Logic  AllPortsSameDT=off  OutDataTypeStr=boolean
  Unit Delay2 : UnitDelay  SampleTime=-1  HasFrameUpgradeWarning=on
  Out1 : Outport  VectorParamsAs1DForOutWhenUnconnected=off
  wires:
  Logical Operator1/1 -> Out1/1
  Compare To Constant2/1 -> Logical Operator1/2
  Compare To Constant1/1 -> Logical Operator1/1
  In1/1 -> Compare To Constant2/1, Unit Delay2/1
  Unit Delay2/1 -> Compare To Constant1/1

== system PMSM_Demo/Control/Controller/PMSM_CONTROLLER/speed_controller/DISCRETE_PT1_SET/discrete_Integrator_Init/only_rising_edge  ==
  In1 : Inport
  Compare To Constant1 : simulink/Logic and Bit Operations/Compare To Constant  relop===  const=0  OutDataTypeStr=uint8  ZeroCross=off
  Compare To Constant2 : simulink/Logic and Bit Operations/Compare To Constant  relop===  const=1  OutDataTypeStr=uint8  ZeroCross=off
  Logical Operator1 : Logic  AllPortsSameDT=off  OutDataTypeStr=boolean
  Unit Delay2 : UnitDelay  SampleTime=-1  HasFrameUpgradeWarning=on
  Out1 : Outport  VectorParamsAs1DForOutWhenUnconnected=off
  wires:
  Unit Delay2/1 -> Compare To Constant1/1
  In1/1 -> Unit Delay2/1, Compare To Constant2/1
  Compare To Constant1/1 -> Logical Operator1/1
  Compare To Constant2/1 -> Logical Operator1/2
  Logical Operator1/1 -> Out1/1

== system PMSM_Demo/Control/Controller/PMSM_CONTROLLER/v_set_source_SW/Calc_Angle/DISCRETE_INTEGRATOR/only_rising_edge  ==
  In1 : Inport
  Compare To Constant1 : simulink/Logic and Bit Operations/Compare To Constant  relop===  const=0  OutDataTypeStr=uint8  ZeroCross=off
  Compare To Constant2 : simulink/Logic and Bit Operations/Compare To Constant  relop===  const=1  OutDataTypeStr=uint8  ZeroCross=off
  Logical Operator1 : Logic  AllPortsSameDT=off  OutDataTypeStr=boolean
  Unit Delay2 : UnitDelay  SampleTime=-1  HasFrameUpgradeWarning=on
  Out1 : Outport  VectorParamsAs1DForOutWhenUnconnected=off
  wires:
  Logical Operator1/1 -> Out1/1
  Compare To Constant2/1 -> Logical Operator1/2
  Compare To Constant1/1 -> Logical Operator1/1
  In1/1 -> Compare To Constant2/1, Unit Delay2/1
  Unit Delay2/1 -> Compare To Constant1/1
